simulink subsystem "HEVIPSSSC"  (R2023a)
settings: Solver=VariableStepAuto  StartTime=0.0  StopTime=10.0  RelTol=1e-3
undefined symbols (not defined in the file): EM1, EM2, PlntHevIpsP1CarrDamp, PlntHevIpsP1PlanetDamp, PlntHevIpsP1RingDamp, PlntHevIpsP1SunDamp, PlntHevIpsP1SunRingRatio, PlntHevIpsP2InDamp, PlntHevIpsP2OutDamp
libraries: fl_lib x16, nesl_utility_internal x3, sdl_lib x2
settings Model: Creator=The MathWorks, Inc.  LastModifiedBy=The MathWorks, Inc.
settings OptimizationCC: ReuseModelBlockBuffer=off

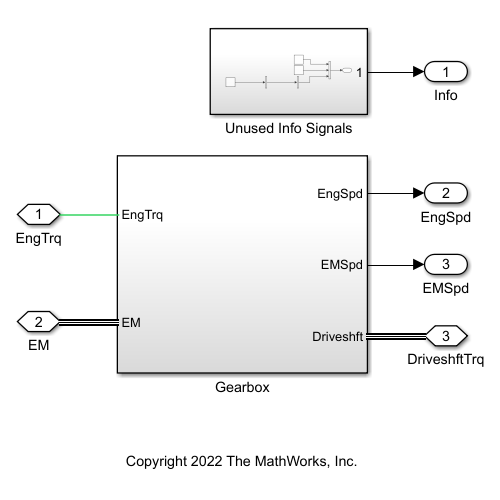
[thumbnail: Simulink's stored preview of the top-level diagram]
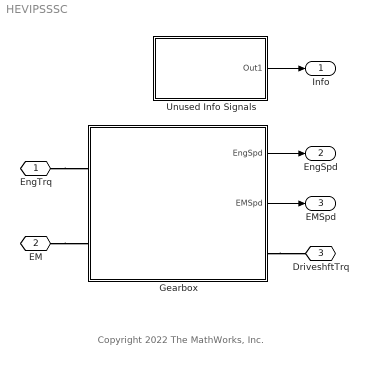
== system HEVIPSSSC ==
  note: Copyright 2022 The MathWorks, Inc.
  Gearbox : Subsystem  VariantControl=Simscape
  Unused Info Signals : Subsystem
  EngTrq : PMIOPort  Side=Left
  EM : PMIOPort  Port=2  Side=Left
  DriveshftTrq : PMIOPort  Port=3  Side=Right
  Info : Outport  VectorParamsAs1DForOutWhenUnconnected=off  BusOutputAsStruct=on
  EngSpd : Outport  Port=2  VectorParamsAs1DForOutWhenUnconnected=off  BusOutputAsStruct=on
  EMSpd : Outport  Port=3  VectorParamsAs1DForOutWhenUnconnected=off  BusOutputAsStruct=on
  wires:
  Gearbox/2(EMSpd) -> EMSpd/1
  Gearbox/1(EngSpd) -> EngSpd/1
  Unused Info Signals/1(Out1) -> Info/1
  connections:
  EM/RConn1 -- Gearbox/LConn2
  Gearbox/RConn1 -- DriveshftTrq/RConn1
  EngTrq/RConn1 -- Gearbox/LConn1

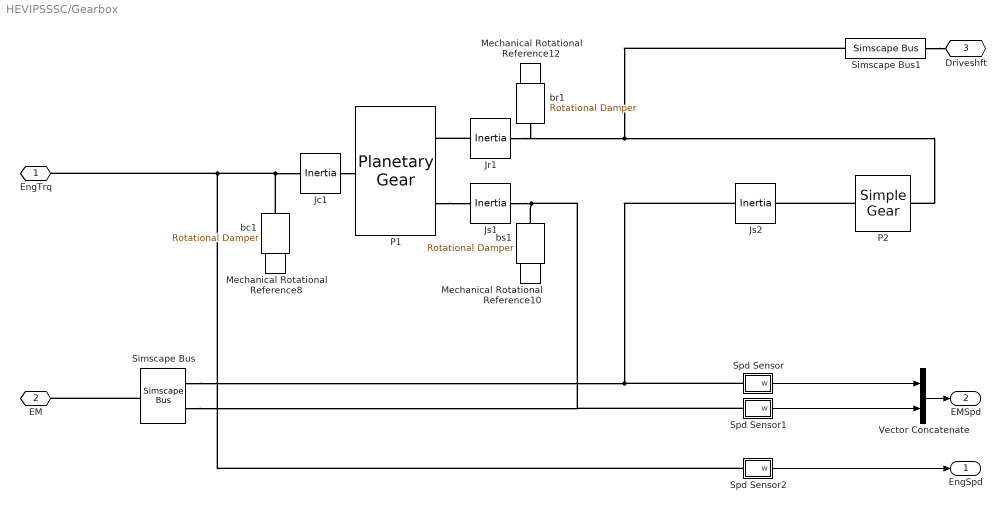
== system HEVIPSSSC/Gearbox ==
  Jc1 : fl_lib/Mechanical/Rotational Elements/Inertia  inertia=PlntHevIpsP1CarrInertia kg*m^2  num_ports=foundation.enum.numPorts2.two  w_specify=on  w_priority=High  w=0 rad/s  w_nominal_specify=off  w_nominal_unit=rad/s  w_nominal_value=1  t_specify=off  t_priority=None  t=0 N*m  t_nominal_specify=off  t_nominal_unit=N*m  t_nominal_value=1
      settings: SourceProductName=Foundation Library  InternalSimscapePortConfiguration="{\"Bottom\":[],\"Left\":[{\"id\":\"I\",\"label\":\"\",\"type\":\"foundation.mechanical.rotational.rotational\"}],\"Right\":[{\"id\":\"J\",\"label\":\"\",\"type\":\"foundation.mechanical.rotational.rotational\"}],\"Top\":[]}"
  Jr1 : fl_lib/Mechanical/Rotational Elements/Inertia  inertia=PlntHevIpsP1RingInertia kg*m^2  num_ports=foundation.enum.numPorts2.two  w_specify=on  w_priority=High  w=0 rad/s  w_nominal_specify=off  w_nominal_unit=rad/s  w_nominal_value=1  t_specify=off  t_priority=None  t=0 N*m  t_nominal_specify=off  t_nominal_unit=N*m  t_nominal_value=1
      settings: SourceProductName=Foundation Library  InternalSimscapePortConfiguration="{\"Bottom\":[],\"Left\":[{\"id\":\"I\",\"label\":\"\",\"type\":\"foundation.mechanical.rotational.rotational\"}],\"Right\":[{\"id\":\"J\",\"label\":\"\",\"type\":\"foundation.mechanical.rotational.rotational\"}],\"Top\":[]}"
  Js1 : fl_lib/Mechanical/Rotational Elements/Inertia  inertia=PlntHevIpsP1SunInertia kg*m^2  num_ports=foundation.enum.numPorts2.two  w_specify=on  w_priority=High  w=0 rad/s  w_nominal_specify=off  w_nominal_unit=rad/s  w_nominal_value=1  t_specify=off  t_priority=None  t=0 N*m  t_nominal_specify=off  t_nominal_unit=N*m  t_nominal_value=1
      settings: SourceProductName=Foundation Library  InternalSimscapePortConfiguration="{\"Bottom\":[],\"Left\":[{\"id\":\"I\",\"label\":\"\",\"type\":\"foundation.mechanical.rotational.rotational\"}],\"Right\":[{\"id\":\"J\",\"label\":\"\",\"type\":\"foundation.mechanical.rotational.rotational\"}],\"Top\":[]}"
  Js2 : fl_lib/Mechanical/Rotational Elements/Inertia  inertia=PlntHevIpsP2InInertia kg*m^2  num_ports=foundation.enum.numPorts2.two  w_specify=on  w_priority=High  w=0 rad/s  w_nominal_specify=off  w_nominal_unit=rad/s  w_nominal_value=1  t_specify=off  t_priority=None  t=0 N*m  t_nominal_specify=off  t_nominal_unit=N*m  t_nominal_value=1
      settings: SourceProductName=Foundation Library  InternalSimscapePortConfiguration="{\"Bottom\":[],\"Left\":[{\"id\":\"I\",\"label\":\"\",\"type\":\"foundation.mechanical.rotational.rotational\"}],\"Right\":[{\"id\":\"J\",\"label\":\"\",\"type\":\"foundation.mechanical.rotational.rotational\"}],\"Top\":[]}"
  Mechanical Rotational Reference10 : fl_lib/Mechanical/Rotational Elements/Mechanical Rotational Reference
      settings: SourceProductName=Foundation Library
  Mechanical Rotational Reference12 : fl_lib/Mechanical/Rotational Elements/Mechanical Rotational Reference
      settings: SourceProductName=Foundation Library
  Mechanical Rotational Reference8 : fl_lib/Mechanical/Rotational Elements/Mechanical Rotational Reference
      settings: SourceProductName=Foundation Library
  P1 : sdl_lib/Gears/Planetary Gear  rs_ratio=1/PlntHevIpsP1SunRingRatio  friction_model=sdl.enum.gear_friction.constant  efficiency=PlntHevIpsP1GearEff  temperature_TLU=[ 280 300 320 ] K  efficiency_sp_TLU=[ 0.95 0.9 0.85 ]  efficiency_rp_TLU=[ 0.95 0.9 0.85 ]  pwr_thr=PlntHevIpsP1GearPwrThresh W  mu_visc=[0 PlntHevIpsP1PlanetDamp] N*m/(rad/s)  model_inertia=1  planet_inertia=PlntHevIpsP1PlanetInertia kg*m^2  thermal_mass=50 J/K  T_init=300 K
      settings: SourceProductName=Driveline  LogSimulationData=on
  P2 : sdl_lib/Gears/Simple Gear  ratio=PlntHevIpsP2GearRatio  rotation_direction=sdl.enum.shaftOutputDirection.same  friction_model=sdl.enum.gear_efficiencies_load.constant  T_noload=0.1 N*m  T_nom=5 N*m  efficiency_nom=0.8  efficiency=PlntHevIpsP2Eff  temperature_TLU=[280, 300, 320] K  load_TLU=[1, 5, 10] N*m  efficiency_TLU=[.95, .9, .85]  efficiency_TLU2=[.85, .8, .75; .95, .9, .85; .85, .8, .7]  w_thr=0.01 rad/s  pwr_thr=PlntHevIpsP2PwrThresh W  enable_backlash=false  hardstop_model=simscape.enum.hardstop.smooth  backlash_distance=1e-3 mm  r_base=0.1 m  transition=1e-4 mm  backlash_stiffness=1e7 N/m  backlash_damping=1e6 N*s/m  coeff_rest=0.7  v_tol=0.001 m/s  f_tol=0.001 N  mu_visc=[PlntHevIpsP2InDamp, PlntHevIpsP2OutDamp] N*m*s/rad  enable_faults=simscape.enum.onoff.off  efficiency_fault=0.05  external_fault=simscape.enum.onoff.off  temporal_fault=simscape.enum.onoff.off  fault_time=5 s  fault_angles=pi / 12 rad  report_fault=simscape.enum.assert.action.none  thermal_mass=50 J/K  temperature_specify=off  temperature_priority=High  temperature=300 K  temperature_nominal_specify=off  temperature_nominal_unit=K  temperature_nominal_value=1  x_backlash_specify=off  x_backlash_priority=None  x_backlash=0 mm  x_backlash_nominal_specify=off  x_backlash_nominal_unit=mm  x_backlash_nominal_value=1  f_hardstop_specify=off  f_hardstop_priority=None  f_hardstop=0 N  f_hardstop_nominal_specify=off  f_hardstop_nominal_unit=N  f_hardstop_nominal_value=1  v_backlash_specify=off  v_backlash_priority=None  v_backlash=0 m/s  v_backlash_nominal_specify=off  v_backlash_nominal_unit=m/s  v_backlash_nominal_value=1
      settings: SourceProductName=Driveline
  Simscape Bus : SimscapeBus  HierarchyStrings=EM1;EM2
  Simscape Bus1 : SimscapeBus  HierarchyStrings=DriveshftTrq1
  Spd Sensor : Subsystem
  Spd Sensor1 : Subsystem
  Spd Sensor2 : Subsystem
  Vector Concatenate : Concatenate
  bc1 : fl_lib/Mechanical/Rotational Elements/Rotational Damper  D=PlntHevIpsP1CarrDamp N*m/(rad/s)  w_specify=on  w_priority=High  w=0 rad/s  w_nominal_specify=off  w_nominal_unit=rad/s  w_nominal_value=1  t_specify=off  t_priority=None  t=0 N*m  t_nominal_specify=off  t_nominal_unit=N*m  t_nominal_value=1
      settings: SourceProductName=Foundation Library
  br1 : fl_lib/Mechanical/Rotational Elements/Rotational Damper  D=PlntHevIpsP1RingDamp N*m/(rad/s)  w_specify=on  w_priority=High  w=0 rad/s  w_nominal_specify=off  w_nominal_unit=rad/s  w_nominal_value=1  t_specify=off  t_priority=None  t=0 N*m  t_nominal_specify=off  t_nominal_unit=N*m  t_nominal_value=1
      settings: SourceProductName=Foundation Library
  bs1 : fl_lib/Mechanical/Rotational Elements/Rotational Damper  D=PlntHevIpsP1SunDamp N*m/(rad/s)  w_specify=on  w_priority=High  w=0 rad/s  w_nominal_specify=off  w_nominal_unit=rad/s  w_nominal_value=1  t_specify=off  t_priority=None  t=0 N*m  t_nominal_specify=off  t_nominal_unit=N*m  t_nominal_value=1
      settings: SourceProductName=Foundation Library
  EngTrq : PMIOPort  Side=Left
  EM : PMIOPort  Port=2  Side=Left
  Driveshft : PMIOPort  Port=3  Side=Right
  EngSpd : Outport  VectorParamsAs1DForOutWhenUnconnected=off
  EMSpd : Outport  Port=2  VectorParamsAs1DForOutWhenUnconnected=off
  wires:
  Spd Sensor2/1(w) -> EngSpd/1
  Spd Sensor1/1(w) -> Vector Concatenate/2
  Spd Sensor/1(w) -> Vector Concatenate/1
  Vector Concatenate/1 -> EMSpd/1
  connections:
  bc1/LConn1 -- Mechanical Rotational Reference8/LConn1
  bs1/LConn1 -- Mechanical Rotational Reference10/LConn1
  br1/LConn1 -- Mechanical Rotational Reference12/LConn1
  P1/RConn2 -- Js1/RConn1
  bc1/RConn1 -- EngTrq/RConn1 -- Spd Sensor2/LConn1 -- Jc1/RConn1
  P2/LConn1 -- Js2/LConn1
  Jr1/RConn1 -- P1/RConn1
  Simscape Bus/RConn1 -- EM/RConn1
  Simscape Bus1/RConn1 -- Driveshft/RConn1
  Js2/RConn1 -- Spd Sensor/LConn1 -- Simscape Bus/LConn1
  Js1/LConn1 -- Simscape Bus/LConn2 -- Spd Sensor1/LConn1 -- bs1/RConn1
  Simscape Bus1/LConn1 -- P2/RConn1 -- Jr1/LConn1 -- br1/RConn1
  Jc1/LConn1 -- P1/LConn1

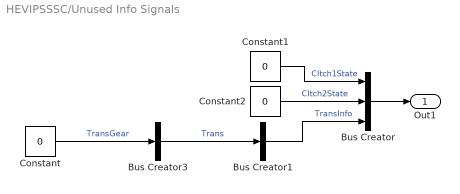
== system HEVIPSSSC/Unused Info Signals ==
  Bus Creator : BusCreator  Inputs=3
  Bus Creator1 : BusCreator  Inputs=1
  Bus Creator3 : BusCreator  Inputs=1
  Constant : Constant  Value=0  SampleTime=-1
  Constant1 : Constant  Value=0  SampleTime=-1
  Constant2 : Constant  Value=0  SampleTime=-1
  Out1 : Outport
  wires:
  Constant2/1 -> Bus Creator/2  "Cltch2State"
  Constant1/1 -> Bus Creator/1  "Cltch1State"
  Bus Creator3/1 -> Bus Creator1/1  "Trans"
  Constant/1 -> Bus Creator3/1  "TransGear"
  Bus Creator/1 -> Out1/1
  Bus Creator1/1 -> Bus Creator/3  "TransInfo"

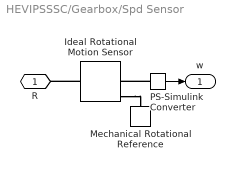
== system HEVIPSSSC/Gearbox/Spd Sensor ==
  Ideal Rotational Motion Sensor : fl_lib/Mechanical/Mechanical Sensors/Ideal Rotational Motion Sensor  reference=foundation.enum.MeasurementReference.difference  acceleration_port=false  velocity_port=true  position_port=true  wrap_angle=simscape.enum.onoff.off  offset=0 rad
      settings: SourceProductName=Foundation Library
  Mechanical Rotational Reference : fl_lib/Mechanical/Rotational Elements/Mechanical Rotational Reference
      settings: SourceProductName=Foundation Library
  PS-Simulink Converter : nesl_utility_internal/PS-Simulink Converter  PhysicalDomain=network_engine_domain  SubClassName=ps_output  LeftPortType=input  RightPortType=output  PseudoPeriodic=off  Frequencies=[]  VectorFormat=inherit  Unit=inherit  AffineConversion=off
  R : PMIOPort  Side=Left
  w : Outport
  wires:
  PS-Simulink Converter/1 -> w/1
  connections:
  Ideal Rotational Motion Sensor/RConn1 -- Mechanical Rotational Reference/LConn1
  Ideal Rotational Motion Sensor/LConn1 -- R/RConn1
  PS-Simulink Converter/LConn1 -- Ideal Rotational Motion Sensor/RConn2

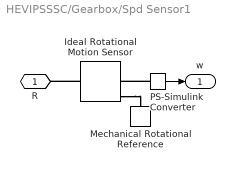
== system HEVIPSSSC/Gearbox/Spd Sensor1 ==
  Ideal Rotational Motion Sensor : fl_lib/Mechanical/Mechanical Sensors/Ideal Rotational Motion Sensor  reference=foundation.enum.MeasurementReference.difference  acceleration_port=false  velocity_port=true  position_port=true  wrap_angle=simscape.enum.onoff.off  offset=0 rad
      settings: SourceProductName=Foundation Library
  Mechanical Rotational Reference : fl_lib/Mechanical/Rotational Elements/Mechanical Rotational Reference
      settings: SourceProductName=Foundation Library
  PS-Simulink Converter : nesl_utility_internal/PS-Simulink Converter  PhysicalDomain=network_engine_domain  SubClassName=ps_output  LeftPortType=input  RightPortType=output  PseudoPeriodic=off  Frequencies=[]  VectorFormat=inherit  Unit=inherit  AffineConversion=off
  R : PMIOPort  Side=Left
  w : Outport
  wires:
  PS-Simulink Converter/1 -> w/1
  connections:
  PS-Simulink Converter/LConn1 -- Ideal Rotational Motion Sensor/RConn2
  Ideal Rotational Motion Sensor/LConn1 -- R/RConn1
  Ideal Rotational Motion Sensor/RConn1 -- Mechanical Rotational Reference/LConn1

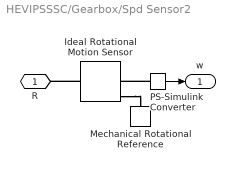
== system HEVIPSSSC/Gearbox/Spd Sensor2 ==
  Ideal Rotational Motion Sensor : fl_lib/Mechanical/Mechanical Sensors/Ideal Rotational Motion Sensor  reference=foundation.enum.MeasurementReference.difference  acceleration_port=false  velocity_port=true  position_port=true  wrap_angle=simscape.enum.onoff.off  offset=0 rad
      settings: SourceProductName=Foundation Library
  Mechanical Rotational Reference : fl_lib/Mechanical/Rotational Elements/Mechanical Rotational Reference
      settings: SourceProductName=Foundation Library
  PS-Simulink Converter : nesl_utility_internal/PS-Simulink Converter  PhysicalDomain=network_engine_domain  SubClassName=ps_output  LeftPortType=input  RightPortType=output  PseudoPeriodic=off  Frequencies=[]  VectorFormat=inherit  Unit=inherit  AffineConversion=off
  R : PMIOPort  Side=Left
  w : Outport
  wires:
  PS-Simulink Converter/1 -> w/1
  connections:
  Ideal Rotational Motion Sensor/RConn1 -- Mechanical Rotational Reference/LConn1
  Ideal Rotational Motion Sensor/LConn1 -- R/RConn1
  PS-Simulink Converter/LConn1 -- Ideal Rotational Motion Sensor/RConn2
